simulink model "model_am_FOC"  (R2025a)
settings: Solver=ode3  StartTime=0.0  StopTime=2  FixedStep=0.0002  RelTol=1e-5  EnableMultiTasking=on
values from neighbouring files (symbols this model uses):
  I = 2.47    [parametres_AM.m]
  i2mN = i2mN2    [parametres_AM.m]
  J = 0.00096 * 5    (= 0.0048)    [parametres_AM.m]
  KI = R1 / (2 * sig * T1 * Kt)    (= 16.5280607989)    [parametres_AM.m]
  KrI = T2 / (2 * 2 * sig * T1)    (= 7.91437626335)    [parametres_AM.m]
  Krw = (J * (1 + sig2)) / (6 * sig * T1 * p^2 * Lh * i2mN)    [parametres_AM.m]
  Kt = 40    [parametres_AM.m]
  L1 = Lh + L1sig    (= 0.579)    [parametres_AM.m]
  L2 = L1    (= 0.579)    [parametres_AM.m]
  Lh = 0.56    [parametres_AM.m]
  M = 3.7    [parametres_AM.m]
  p = 2    [parametres_AM.m]
  R1 = 7.03    [parametres_AM.m]
  R2 = 3.44    [parametres_AM.m]
  sig = 1 - (Lh^2 / (L1 * L2))    (= 0.0645535599763)    [parametres_AM.m]
  T1 = L1 / R1    (= 0.0823613086771)    [parametres_AM.m]
  T2 = L2 / R2    (= 0.168313953488)    [parametres_AM.m]
  TiI = TrI / KrI    (= 0.0212668627176)    [parametres_AM.m]
  Tiw = Trw / Krw    [parametres_AM.m]
  Ulim = 380    [parametres_AM.m]
undefined symbols (not defined in the file or in its folder): sigbuilder_block
settings Model: Creator=Kajo  LastModifiedBy=emaka
settings SolverCC: AlgebraicLoopSolver=TrustRegion
settings DataIOCC: LimitDataPoints=on  SaveFormat=Array  SignalLoggingSaveFormat=ModelDataLogs  ReturnWorkspaceOutputs=off
settings OptimizationCC: ExpressionDepthLimit=2147483647.0  LifeSpan=inf
settings DebuggingCC: UnderspecifiedInitializationDetection=Classic  MergeDetectMultiDrivingBlocksExec=none  SolverPrmCheckMsg=warning  FcnCallInpInsideContextMsg=warning  UnconnectedInputMsg=warning  UnconnectedOutputMsg=warning  UnconnectedLineMsg=warning  StateNameClashWarn=warning  SFUnexpectedBacktrackingDiag=warning  SFNoUnconditionalDefaultTransitionDiag=warning  SFExecutionAtInitializationDiag=none  ArithmeticOperatorsInVariantConditions=warning
settings HardwareCC: ProdBitPerPointer=32.0  ProdBitPerSizeT=32.0  ProdBitPerPtrDiffT=32.0  ProdLargestAtomicFloat=None  ProdIntDivRoundTo=Undefined  ProdEndianess=Unspecified  ProdWordSize=32.0  ProdHWDeviceType=32-bit Generic
settings ModelReferenceCC: EnableRefExpFcnMdlSchedulingChecks=on  PropagateSignalLabelsOutOfModel=off
settings SFSimCC: SimUseLocalCustomCode=off  CustomCodeUndefinedFunction=UseInterfaceOnly
settings RTWCC: RTWUseLocalCustomCode=off  GPUComputeCapability=3.5
settings CodeAppCC: StateflowObjectComments=on
settings GRTTargetCC: TargetLangStandard=C89/C90 (ANSI)  CombineOutputUpdateFcns=off  GRTInterface=on
settings ConfigComp: CovMetricSettings=dw  CovSaveCumulativeToWorkspaceVar=on  CovSaveSingleToWorkspaceVar=on  CovExternalEMLEnable=off  CovSFcnEnable=off

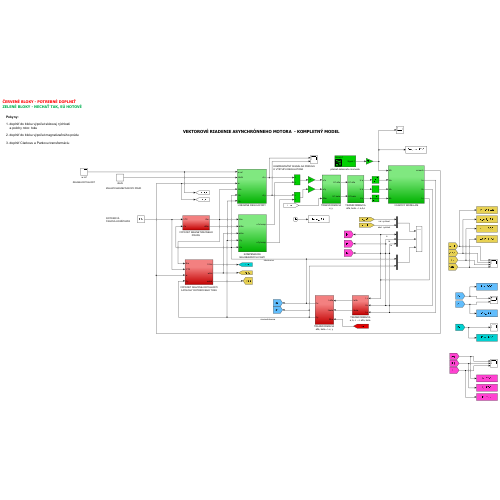
[thumbnail: Simulink's stored preview of the top-level diagram]
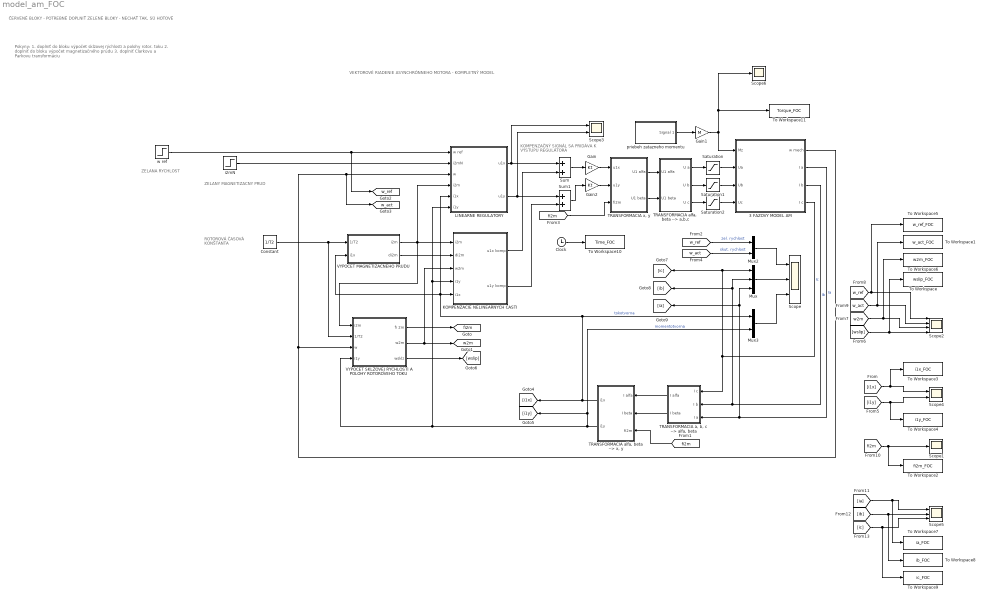
== system model_am_FOC ==
  note: Pokyny:
      |
      | 1. doplniť do bloku výpočet sklzovej rýchlosti
      | a polohy rotor. toku
      |
      | 2. doplniť do bloku výpočet magnetizačného prúdu
      |
      | 3. doplniť Clarkovu a Parkovu transformáciu
  note: ZELANA RYCHLOST
  note: KOMPENZAČNÝ SIGNÁL SA PRIDÁVA
      | K VÝSTUPU REGULÁTORA
  note: ROTOROVÁ
      | ČASOVÁ KONŠTANTA
  note: ČERVENÉ BLOKY - POTREBNÉ DOPLNIŤ
      | ZELENÉ BLOKY - NECHAŤ TAK, SÚ HOTOVÉ
  note: VEKTOROVÉ RIADENIE ASYNCHRÓNNEHO MOTORA - KOMPLETNÝ MODEL
  note: ZELANY MAGNETIZACNY PRUD
  3 FAZOVY MODEL AM : Subsystem
  Clock : Clock
  Constant : Constant  Value=1/T2
  Gain : Gain  Gain=Kt
  Gain1 : Gain  Gain=M
  Gain2 : Gain  Gain=Kt
  KOMPENZACIE NELINEARNYCH CASTI : Subsystem
  LINEARNE REGULATORY : Subsystem
  Mux : Mux  Inputs=3
  Mux2 : Mux  Inputs=2
  Mux3 : Mux  Inputs=2
  Saturation : Saturate  UpperLimit=Ulim  LowerLimit=-Ulim
  Saturation1 : Saturate  UpperLimit=Ulim  LowerLimit=-Ulim
  Saturation2 : Saturate  UpperLimit=Ulim  LowerLimit=-Ulim
  Scope : Scope  NumInputPorts=3
      settings: ActiveDisplayYMinimum=-13.916341130679911  ActiveDisplayYMaximum=125.24707017611922
  Scope1 : Scope
      settings: ActiveDisplayYMinimum=-1  ActiveDisplayYMaximum=1
  Scope2 : Scope  NumInputPorts=4
      settings: ActiveDisplayYMinimum=-1  ActiveDisplayYMaximum=1  DataLoggingVariableName=ScopeData3
  Scope3 : Scope  NumInputPorts=2
      settings: ActiveDisplayYMinimum=-0.016508812303007426  ActiveDisplayYMaximum=0.14857931072706687  DataLoggingVariableName=ScopeData4
  Scope4 : Scope  NumInputPorts=2
      settings: ActiveDisplayYMinimum=-1  ActiveDisplayYMaximum=1  DataLoggingVariableName=ScopeData5
  Scope5 : Scope  NumInputPorts=3
      settings: ActiveDisplayYMinimum=-1  ActiveDisplayYMaximum=1  DataLoggingVariableName=ScopeData6
  Scope6 : Scope
      settings: ActiveDisplayYMinimum=-1  ActiveDisplayYMaximum=1  DataLoggingVariableName=ScopeData7
  Sum : Sum
  Sum1 : Sum
  "TRANSFORMACIA a, b, c  --> alfa, beta " : Subsystem
  "TRANSFORMACIA alfa, beta --> a,b,c" : Subsystem
  "TRANSFORMACIA alfa, beta --> x, y" : Subsystem
  "TRANSFORMACIA x, y " : Subsystem
  To Workspace : ToWorkspace  VariableName=wslip_FOC  SampleTime=-1
  To Workspace1 : ToWorkspace  VariableName=w_act_FOC  SampleTime=-1
  To Workspace10 : ToWorkspace  VariableName=Time_FOC  SampleTime=-1
  To Workspace11 : ToWorkspace  VariableName=Torque_FOC  SampleTime=-1
  To Workspace2 : ToWorkspace  VariableName=fi2m_FOC  SampleTime=-1
  To Workspace3 : ToWorkspace  VariableName=i1x_FOC  SampleTime=-1
  To Workspace4 : ToWorkspace  VariableName=i1y_FOC  SampleTime=-1
  To Workspace5 : ToWorkspace  VariableName=w_ref_FOC  SampleTime=-1
  To Workspace6 : ToWorkspace  VariableName=w2m_FOC  SampleTime=-1
  To Workspace7 : ToWorkspace  VariableName=ia_FOC  SampleTime=-1
  To Workspace8 : ToWorkspace  VariableName=ib_FOC  SampleTime=-1
  To Workspace9 : ToWorkspace  VariableName=ic_FOC  SampleTime=-1
  VYPOCET MAGNETIZACNEHO PRUDU : Subsystem
  VYPOCET SKLZOVEJ RYCHLOSTI A POLOHY ROTOROVEHO TOKU : Subsystem
  i2mN : Step  Time=0  After=i2mN  SampleTime=0
  priebeh zatazneho momentu : Subsystem  Tag=STV Subsys  LoadFcn=sigbuilder_block('load');  StartFcn=sigbuilder_block('start');  StopFcn=sigbuilder_block('stop');  ClipboardFcn=sigbuilder_block('clipboard');  mask(Sigbuilder block){tuvar=[0:10]}
      mask help: Simulink:masks:SigbuilderBlock_MD
      mask init:
      | if ~strcmp(get_param(bdroot(gcbh),'SimulationStatus'),'stopped') tuvar = sigbuilder_block('maskInit'); end
      settings: CopyFcn=sigbuilder_block('copy');  DeleteFcn=sigbuilder_block('delete');  ModelCloseFcn=sigbuilder_block('modelClose');  PreSaveFcn=sigbuilder_block('preSave');  PauseFcn=sigbuilder_block('pause');  ContinueFcn=sigbuilder_block('continue');  NameChangeFcn=sigbuilder_block('namechange');  OpenFcn=sigbuilder_block('open',[436.5 297.75 1045.5 630 ]);  CloseFcn=sigbuilder_block('close');
      mask Display: plot(0, 0, 100, 100,[2, 2, 32, 32, 2], [68, 8, 8, 68, 68],[32, 2], [38, 38], [32, 19, 2],[53, 60, 44], [32, 17, 17, 2],[16, 16, 31, 31]);txt = getActiveGroup(gcbh);text(2, 100, txt,'verticalAlignment', 'top');
  w ref : Step  Time=0.4  After=70  SampleTime=0
  tag scope: fi2m=global, w2m=global, w_act=global, w_ref=global
  wires:
  priebeh zatazneho momentu/1(Signal 1) -> Gain1/1
  Gain1/1 -> 3 FAZOVY MODEL AM/1(Mz), Scope6/1, To Workspace11/1
  LINEARNE REGULATORY/1(u1x) -> Sum/1, Scope3/1
  LINEARNE REGULATORY/2(u1y) -> Scope3/2, Sum1/1
  KOMPENZACIE NELINEARNYCH CASTI/1(u1x komp) -> Sum/2
  KOMPENZACIE NELINEARNYCH CASTI/2(u1y komp) -> Sum1/2
  "TRANSFORMACIA a, b, c  --> alfa, beta "/1(I alfa) -> "TRANSFORMACIA alfa, beta --> x, y"/1(I alfa)
  "TRANSFORMACIA a, b, c  --> alfa, beta "/2(I beta) -> "TRANSFORMACIA alfa, beta --> x, y"/2(I beta)
  3 FAZOVY MODEL AM/1(w mech) -> [w_act], LINEARNE REGULATORY/3(w), VYPOCET SKLZOVEJ RYCHLOSTI A POLOHY ROTOROVEHO TOKU/3(w)
  i2mN/1 -> LINEARNE REGULATORY/2(i2mN)
  3 FAZOVY MODEL AM/4(I c) -> Mux/1, [ic], "TRANSFORMACIA a, b, c  --> alfa, beta "/1(I c)  "Ic"
  3 FAZOVY MODEL AM/3(I b) -> Mux/2, [ib], "TRANSFORMACIA a, b, c  --> alfa, beta "/2(I b)  "Ib"
  3 FAZOVY MODEL AM/2(I a) -> [ia], Mux/3, "TRANSFORMACIA a, b, c  --> alfa, beta "/3(I a)  "Ia"
  Constant/1 -> VYPOCET SKLZOVEJ RYCHLOSTI A POLOHY ROTOROVEHO TOKU/2(1/T2), VYPOCET MAGNETIZACNEHO PRUDU/1(1/T2)
  VYPOCET MAGNETIZACNEHO PRUDU/1(i2m) -> LINEARNE REGULATORY/4(i2m), VYPOCET SKLZOVEJ RYCHLOSTI A POLOHY ROTOROVEHO TOKU/1(i2m), KOMPENZACIE NELINEARNYCH CASTI/1(i2m)
  VYPOCET MAGNETIZACNEHO PRUDU/2(di2m) -> KOMPENZACIE NELINEARNYCH CASTI/2(di2m)
  Gain/1 -> "TRANSFORMACIA x, y "/1(u1x)
  Gain2/1 -> "TRANSFORMACIA x, y "/2(u1y)
  "TRANSFORMACIA x, y "/1(U1 alfa) -> "TRANSFORMACIA alfa, beta --> a,b,c"/1(U1 alfa)
  "TRANSFORMACIA x, y "/2(U1 beta) -> "TRANSFORMACIA alfa, beta --> a,b,c"/2(U1 beta)
  "TRANSFORMACIA alfa, beta --> a,b,c"/1(U a) -> Saturation/1
  "TRANSFORMACIA alfa, beta --> a,b,c"/2(U b) -> Saturation1/1
  "TRANSFORMACIA alfa, beta --> a,b,c"/3(U c) -> Saturation2/1
  Saturation/1 -> 3 FAZOVY MODEL AM/2(Ua)
  Saturation1/1 -> 3 FAZOVY MODEL AM/3(Ub)
  Saturation2/1 -> 3 FAZOVY MODEL AM/4(Uc)
  Sum/1 -> Gain/1
  Sum1/1 -> Gain2/1
  "TRANSFORMACIA alfa, beta --> x, y"/2(i1y) -> [i1y], Mux3/2, KOMPENZACIE NELINEARNYCH CASTI/4(i1y), LINEARNE REGULATORY/6(i1y), VYPOCET SKLZOVEJ RYCHLOSTI A POLOHY ROTOROVEHO TOKU/4(i1y)  "momentotvorna"
  VYPOCET SKLZOVEJ RYCHLOSTI A POLOHY ROTOROVEHO TOKU/2(w2m) -> KOMPENZACIE NELINEARNYCH CASTI/3(w2m), [w2m]
  "TRANSFORMACIA alfa, beta --> x, y"/1(i1x) -> [i1x], LINEARNE REGULATORY/5(i1x), VYPOCET MAGNETIZACNEHO PRUDU/2(i1x), KOMPENZACIE NELINEARNYCH CASTI/5(i1x), Mux3/1  "tokotvorna"
  w ref/1 -> LINEARNE REGULATORY/1(w ref), [w_ref]
  VYPOCET SKLZOVEJ RYCHLOSTI A POLOHY ROTOROVEHO TOKU/1(fi 2m) -> [fi2m]
  [fi2m] -> "TRANSFORMACIA alfa, beta --> x, y"/3(fi2m)
  [fi2m] -> "TRANSFORMACIA x, y "/3("fi2m ")
  Mux2/1 -> Scope/1
  [w_ref] -> Mux2/1  "zel. rychlost"
  [w_act] -> Mux2/2  "skut. rychlost"
  Mux3/1 -> Scope/3
  Mux/1 -> Scope/2
  [i1x] -> To Workspace3/1, Scope4/1
  [i1y] -> To Workspace4/1, Scope4/2
  VYPOCET SKLZOVEJ RYCHLOSTI A POLOHY ROTOROVEHO TOKU/3(wsklz) -> [wslip]
  [wslip] -> To Workspace/1, Scope2/4
  [w2m] -> To Workspace6/1, Scope2/3
  [w_ref] -> To Workspace5/1, Scope2/1
  [w_act] -> To Workspace1/1, Scope2/2
  [fi2m] -> To Workspace2/1, Scope1/1
  [ia] -> To Workspace7/1, Scope5/1
  [ib] -> To Workspace8/1, Scope5/2
  [ic] -> To Workspace9/1, Scope5/3
  Clock/1 -> To Workspace10/1

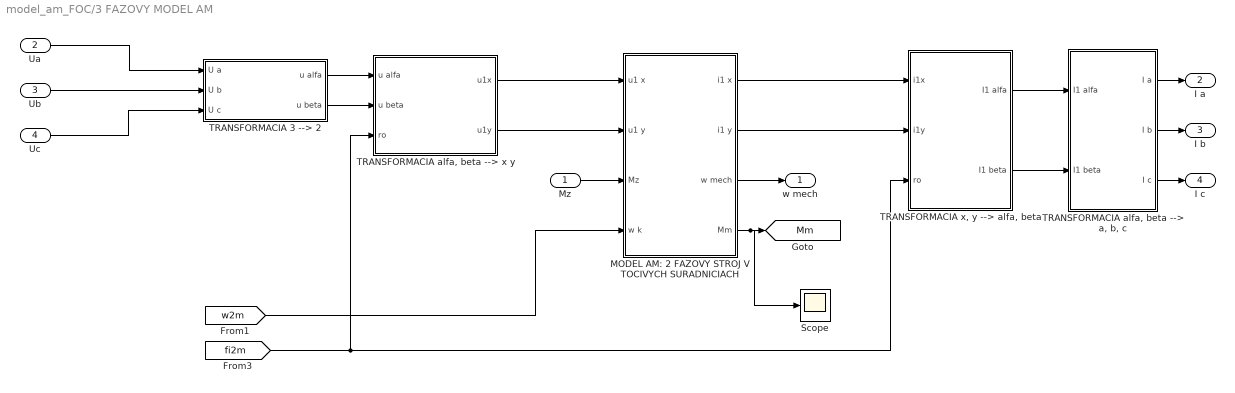
== system model_am_FOC/3 FAZOVY MODEL AM ==
  Mz : Inport
  Ua : Inport  Port=2
  Ub : Inport  Port=3
  Uc : Inport  Port=4
  MODEL AM: 2 FAZOVY STROJ V TOCIVYCH SURADNICIACH : Subsystem
  Scope : Scope
      settings: ActiveDisplayYMinimum=-2.9719517266428888  ActiveDisplayYMaximum=3.6440018137289671  DataLoggingVariableName=ScopeData2
  "TRANSFORMACIA alfa, beta --> x y" : Subsystem
  TRANSFORMACIA 3 --> 2 : Subsystem
  "TRANSFORMACIA alfa, beta --> a, b, c" : Subsystem
  "TRANSFORMACIA x, y --> alfa, beta" : Subsystem
  w mech : Outport  VectorParamsAs1DForOutWhenUnconnected=off
  I a : Outport  Port=2  VectorParamsAs1DForOutWhenUnconnected=off
  I b : Outport  Port=3  VectorParamsAs1DForOutWhenUnconnected=off
  I c : Outport  Port=4  VectorParamsAs1DForOutWhenUnconnected=off
  tag scope: Mm=global
  wires:
  TRANSFORMACIA 3 --> 2/1(u alfa) -> "TRANSFORMACIA alfa, beta --> x y"/1(u alfa)
  TRANSFORMACIA 3 --> 2/2(u beta) -> "TRANSFORMACIA alfa, beta --> x y"/2(u beta)
  "TRANSFORMACIA alfa, beta --> x y"/1(u1x) -> MODEL AM: 2 FAZOVY STROJ V TOCIVYCH SURADNICIACH/1(u1 x)
  "TRANSFORMACIA alfa, beta --> x y"/2(u1y) -> MODEL AM: 2 FAZOVY STROJ V TOCIVYCH SURADNICIACH/2(u1 y)
  "TRANSFORMACIA x, y --> alfa, beta"/1(I1 alfa) -> "TRANSFORMACIA alfa, beta --> a, b, c"/1(I1 alfa)
  "TRANSFORMACIA x, y --> alfa, beta"/2(I1 beta) -> "TRANSFORMACIA alfa, beta --> a, b, c"/2(I1 beta)
  "TRANSFORMACIA alfa, beta --> a, b, c"/1(I a) -> I a/1
  "TRANSFORMACIA alfa, beta --> a, b, c"/2(I b) -> I b/1
  "TRANSFORMACIA alfa, beta --> a, b, c"/3(I c) -> I c/1
  Ua/1 -> TRANSFORMACIA 3 --> 2/1(U a)
  Ub/1 -> TRANSFORMACIA 3 --> 2/2(U b)
  Uc/1 -> TRANSFORMACIA 3 --> 2/3(U c)
  Mz/1 -> MODEL AM: 2 FAZOVY STROJ V TOCIVYCH SURADNICIACH/3(Mz)
  MODEL AM: 2 FAZOVY STROJ V TOCIVYCH SURADNICIACH/1(i1 x) -> "TRANSFORMACIA x, y --> alfa, beta"/1(i1x)
  MODEL AM: 2 FAZOVY STROJ V TOCIVYCH SURADNICIACH/2(i1 y) -> "TRANSFORMACIA x, y --> alfa, beta"/2(i1y)
  MODEL AM: 2 FAZOVY STROJ V TOCIVYCH SURADNICIACH/3(w mech) -> w mech/1
  [fi2m] -> "TRANSFORMACIA x, y --> alfa, beta"/3("ro "), "TRANSFORMACIA alfa, beta --> x y"/3(ro)
  [w2m] -> MODEL AM: 2 FAZOVY STROJ V TOCIVYCH SURADNICIACH/4(w k)
  MODEL AM: 2 FAZOVY STROJ V TOCIVYCH SURADNICIACH/4(Mm) -> Scope/1, [Mm]

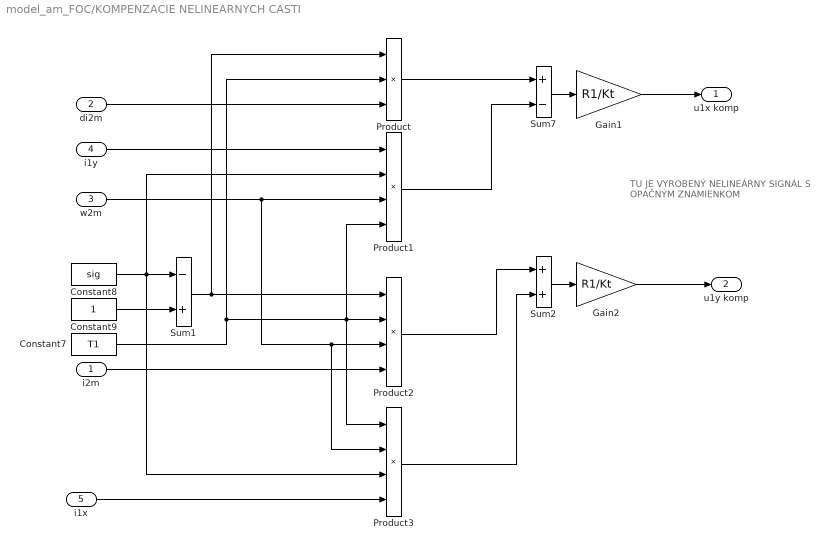
== system model_am_FOC/KOMPENZACIE NELINEARNYCH CASTI ==
  note: TU JE VYROBENÝ NELINEÁRNY SIGNÁL
      | S OPAČNÝM ZNAMIENKOM
  i2m : Inport
  di2m : Inport  Port=2
  w2m : Inport  Port=3
  i1y : Inport  Port=4
  i1x : Inport  Port=5
  Constant7 : Constant  Value=T1
  Constant8 : Constant  Value=sig
  Constant9 : Constant
  Gain1 : Gain  Gain=R1/Kt
  Gain2 : Gain  Gain=R1/Kt
  Product : Product  Inputs=3  RndMeth=Zero
  Product1 : Product  Inputs=4  RndMeth=Zero
  Product2 : Product  Inputs=4  RndMeth=Zero
  Product3 : Product  Inputs=4  RndMeth=Zero
  Sum1 : Sum  Inputs=-+
  Sum2 : Sum
  Sum7 : Sum  Inputs=+-
  u1x komp : Outport  VectorParamsAs1DForOutWhenUnconnected=off
  u1y komp : Outport  Port=2  VectorParamsAs1DForOutWhenUnconnected=off
  wires:
  Sum7/1 -> Gain1/1
  Sum2/1 -> Gain2/1
  Product/1 -> Sum7/1
  Product1/1 -> Sum7/2
  Product2/1 -> Sum2/1
  Product3/1 -> Sum2/2
  Constant9/1 -> Sum1/2
  Sum1/1 -> Product/1, Product2/1
  Constant7/1 -> Product/2, Product2/2, Product1/4, Product3/1
  di2m/1 -> Product/3
  i2m/1 -> Product2/4
  w2m/1 -> Product1/3, Product2/3, Product3/2
  i1y/1 -> Product1/1
  i1x/1 -> Product3/4
  Constant8/1 -> Sum1/1, Product1/2, Product3/3
  Gain1/1 -> u1x komp/1
  Gain2/1 -> u1y komp/1

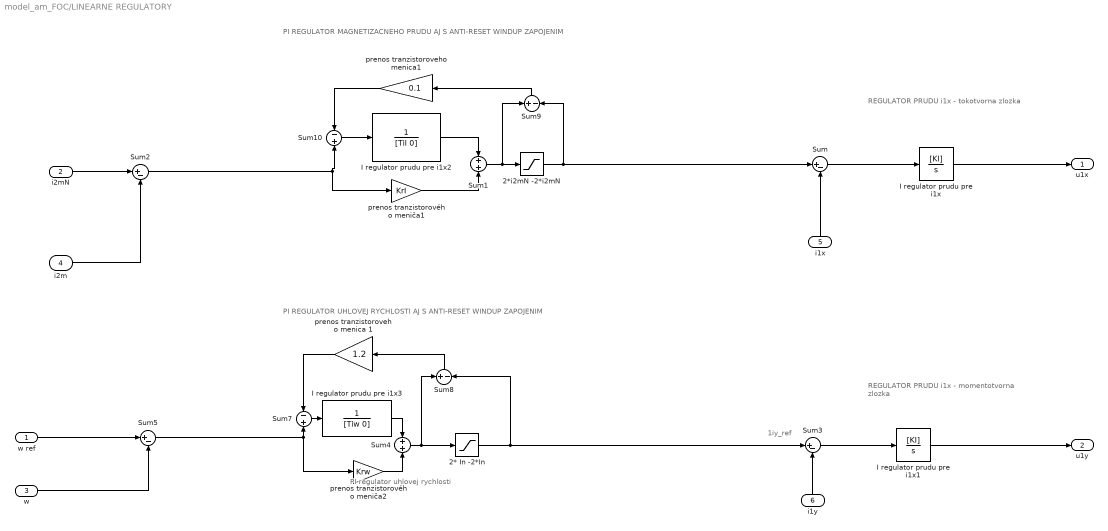
== system model_am_FOC/LINEARNE REGULATORY ==
  note: REGULATOR PRUDU
      | i1x - tokotvorna zlozka
  note: PI REGULATOR MAGNETIZACNEHO PRUDU
      | AJ S ANTI-RESET WINDUP ZAPOJENIM
  note: 1iy_ref
  note: PI regulator
      | uhlovej rychlosti
  note: PI REGULATOR UHLOVEJ RYCHLOSTI
      | AJ S ANTI-RESET WINDUP ZAPOJENIM
  note: REGULATOR PRUDU
      | i1x - momentotvorna zlozka
  w ref : Inport
  i2mN : Inport  Port=2
  w : Inport  Port=3
  i2m : Inport  Port=4
  i1x : Inport  Port=5
  i1y : Inport  Port=6
  2* In -2*In : Saturate  UpperLimit=I*1.5  LowerLimit=-I*1.5
  2*i2mN -2*i2mN : Saturate  UpperLimit=1.5*i2mN  LowerLimit=-1.5*i2mN
  I regulator prudu pre i1x : TransferFcn  Numerator=[KI]  Denominator=[1 0]
  I regulator prudu pre i1x1 : TransferFcn  Numerator=[KI]  Denominator=[1 0]
  I regulator prudu pre i1x2 : TransferFcn  Denominator=[TiI 0]
  I regulator prudu pre i1x3 : TransferFcn  Denominator=[Tiw 0]
  Sum{,2..3,5} (4 alike) : Sum  Inputs=|+-
  Sum1 : Sum
  Sum10 : Sum  Inputs=-+
  Sum4 : Sum
  Sum7 : Sum  Inputs=-+
  Sum8 : Sum  Inputs=+-
  Sum9 : Sum  Inputs=+-
  prenos tranzistoroveho menica 1 : Gain  Gain=1.2
  prenos tranzistoroveho menica1 : Gain  Gain=0.1
  prenos tranzistorového meniča1 : Gain  Gain=KrI
  prenos tranzistorového meniča2 : Gain  Gain=Krw
  u1x : Outport  VectorParamsAs1DForOutWhenUnconnected=off
  u1y : Outport  Port=2  VectorParamsAs1DForOutWhenUnconnected=off
  wires:
  w ref/1 -> Sum5/1
  i1x/1 -> Sum/2
  i1y/1 -> Sum3/2
  w/1 -> Sum5/2
  i2mN/1 -> Sum2/1
  i2m/1 -> Sum2/2
  2* In -2*In/1 -> Sum8/2, Sum3/1
  I regulator prudu pre i1x/1 -> u1x/1
  I regulator prudu pre i1x1/1 -> u1y/1
  Sum/1 -> I regulator prudu pre i1x/1
  Sum3/1 -> I regulator prudu pre i1x1/1
  Sum1/1 -> 2*i2mN -2*i2mN/1, Sum9/1
  Sum9/1 -> prenos tranzistoroveho menica1/1
  Sum2/1 -> prenos tranzistorového meniča1/1, Sum10/2
  prenos tranzistorového meniča1/1 -> Sum1/2
  I regulator prudu pre i1x2/1 -> Sum1/1
  prenos tranzistoroveho menica1/1 -> Sum10/1
  Sum10/1 -> I regulator prudu pre i1x2/1
  2*i2mN -2*i2mN/1 -> Sum/1, Sum9/2
  Sum5/1 -> prenos tranzistorového meniča2/1, Sum7/2
  Sum7/1 -> I regulator prudu pre i1x3/1
  prenos tranzistorového meniča2/1 -> Sum4/2
  I regulator prudu pre i1x3/1 -> Sum4/1
  Sum8/1 -> prenos tranzistoroveho menica 1/1
  Sum4/1 -> 2* In -2*In/1, Sum8/1
  prenos tranzistoroveho menica 1/1 -> Sum7/1

== system model_am_FOC/TRANSFORMACIA a, b, c  --> alfa, beta  ==
  I c : Inport
  I b : Inport  Port=2
  I a : Inport  Port=3
  Gain : Gain  Gain=1/sqrt(3)
  Sum : Sum  Inputs=|+-
  I alfa : Outport  VectorParamsAs1DForOutWhenUnconnected=off
  I beta : Outport  Port=2  VectorParamsAs1DForOutWhenUnconnected=off
  wires:
  I b/1 -> Sum/1
  I c/1 -> Sum/2
  Sum/1 -> Gain/1
  Gain/1 -> I beta/1
  I a/1 -> I alfa/1

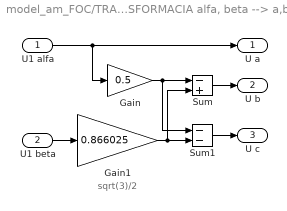
== system model_am_FOC/TRANSFORMACIA alfa, beta --> a,b,c ==
  note: sqrt(3)/2
  U1 alfa : Inport
  U1 beta : Inport  Port=2
  Gain : Gain  Gain=0.5
  Gain1 : Gain  Gain=0.866025
  Sum : Sum  Inputs=-+
  Sum1 : Sum  Inputs=--
  U a : Outport  VectorParamsAs1DForOutWhenUnconnected=off
  U b : Outport  Port=2  VectorParamsAs1DForOutWhenUnconnected=off
  U c : Outport  Port=3  VectorParamsAs1DForOutWhenUnconnected=off
  wires:
  Sum1/1 -> U c/1
  Gain1/1 -> Sum1/2, Sum/2
  U1 beta/1 -> Gain1/1
  Sum/1 -> U b/1
  Gain/1 -> Sum1/1, Sum/1
  U1 alfa/1 -> U a/1, Gain/1

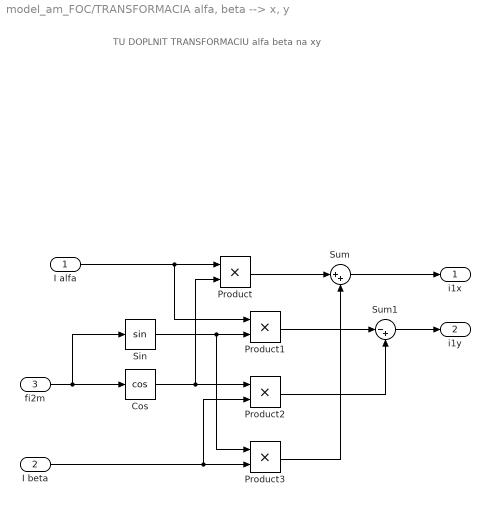
== system model_am_FOC/TRANSFORMACIA alfa, beta --> x, y ==
  note: TU DOPLNIT TRANSFORMACIU
      | alfa beta na xy
  I alfa : Inport
  I beta : Inport  Port=2
  fi2m : Inport  Port=3
  Cos : Trigonometry  Operator=cos
  Product{,1..3} (4 alike) : Product
  Sin : Trigonometry
  Sum : Sum  Inputs=|++
  Sum1 : Sum  Inputs=|-+
  i1x : Outport  VectorParamsAs1DForOutWhenUnconnected=off
  i1y : Outport  Port=2  VectorParamsAs1DForOutWhenUnconnected=off
  wires:
  I alfa/1 -> Product1/1, Product/1
  Product/1 -> Sum/1
  fi2m/1 -> Sin/1, Cos/1
  Sin/1 -> Product3/1, Product1/2
  Cos/1 -> Product2/1, Product/2
  I beta/1 -> Product3/2, Product2/2
  Product3/1 -> Sum/2
  Product1/1 -> Sum1/1
  Sum/1 -> i1x/1
  Sum1/1 -> i1y/1
  Product2/1 -> Sum1/2

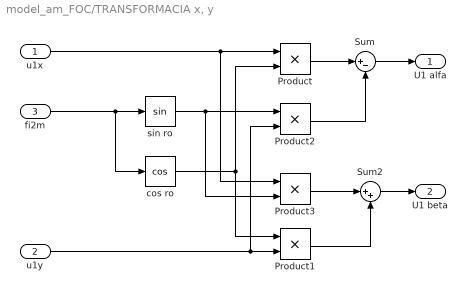
== system model_am_FOC/TRANSFORMACIA x, y  ==
  u1x : Inport
  u1y : Inport  Port=2
  "fi2m " : Inport  Port=3
  Product{,1..3} (4 alike) : Product  RndMeth=Zero
  Sum : Sum  Inputs=|+-
  Sum2 : Sum  Inputs=|++
  cos ro : Trigonometry  Operator=cos
  sin ro : Trigonometry
  U1 alfa : Outport  VectorParamsAs1DForOutWhenUnconnected=off
  U1 beta : Outport  Port=2  VectorParamsAs1DForOutWhenUnconnected=off
  wires:
  Product1/1 -> Sum2/2
  Product3/1 -> Sum2/1
  Product2/1 -> Sum/2
  Product/1 -> Sum/1
  u1y/1 -> Product2/2, Product1/2
  sin ro/1 -> Product3/2, Product2/1
  cos ro/1 -> Product1/1, Product/2
  u1x/1 -> Product/1, Product3/1
  Sum2/1 -> U1 beta/1
  Sum/1 -> U1 alfa/1
  "fi2m "/1 -> cos ro/1, sin ro/1

== system model_am_FOC/VYPOCET MAGNETIZACNEHO PRUDU ==
  note: TU DOPLNIT VYPOCET
      | MAGNETIZACNEHO PRUDU
  1/T2 : Inport
  i1x : Inport  Port=2
  Integrator : Integrator
  Product : Product
  Sum : Sum  Inputs=|+-
  i2m : Outport  VectorParamsAs1DForOutWhenUnconnected=off
  di2m : Outport  Port=2  VectorParamsAs1DForOutWhenUnconnected=off
  wires:
  i1x/1 -> Sum/1
  1/T2/1 -> Product/2
  Product/1 -> di2m/1, Integrator/1
  Sum/1 -> Product/1
  Integrator/1 -> i2m/1, Sum/2

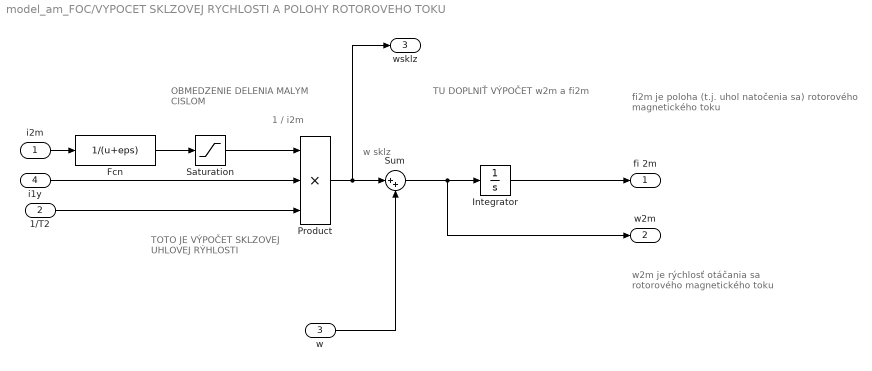
== system model_am_FOC/VYPOCET SKLZOVEJ RYCHLOSTI A POLOHY ROTOROVEHO TOKU ==
  note: TOTO JE VÝPOČET
      | SKLZOVEJ UHLOVEJ RÝHLOSTI
  note: TU DOPLNIŤ
      | VÝPOČET w2m a fi2m
  note: 1 / i2m
  note: w sklz
  note: OBMEDZENIE
      | DELENIA
      | MALYM CISLOM
  note: w2m je rýchlosť
      | otáčania sa rotorového
      | magnetického toku
  note: fi2m je poloha (t.j. uhol natočenia sa) rotorového
      | magnetického toku
  i2m : Inport
  1/T2 : Inport  Port=2
  w : Inport  Port=3
  i1y : Inport  Port=4
  Fcn : Fcn  Expr=1/(u+eps)
  Integrator : Integrator
  Product : Product  Inputs=3  RndMeth=Zero
  Saturation : Saturate  UpperLimit=300  LowerLimit=-300
  Sum : Sum  Inputs=|++
  fi 2m : Outport  VectorParamsAs1DForOutWhenUnconnected=off
  w2m : Outport  Port=2  VectorParamsAs1DForOutWhenUnconnected=off
  wsklz : Outport  Port=3
  wires:
  1/T2/1 -> Product/3
  i2m/1 -> Fcn/1
  Fcn/1 -> Saturation/1
  Product/1 -> wsklz/1, Sum/1
  w/1 -> Sum/2
  Saturation/1 -> Product/1
  i1y/1 -> Product/2
  Sum/1 -> w2m/1, Integrator/1
  Integrator/1 -> fi 2m/1

== system model_am_FOC/priebeh zatazneho momentu ==
  Demux : Demux  Tag=STV Demux  Outputs=1
      settings: DisplayOption=none
  FromWs : FromWorkspace  Tag=STV FromWs  VariableName=tuvar
      SigBuilderData=|
      | common.afterFinalStr = 'Extrapolate'
      | common.sampleTime = 0
      | dataSet.timeRange = [0 5]
      | dataSet.name = 'Group 1'
      | sbobj.Groups.Name = 'Group 1'
      | sbobj.Groups.Signals.Name = 'Signal 1'
      | sbobj.Groups.Signals.XData = [0 1.2 1.2 5]
      | sbobj.Groups.Signals.YData = [0 0 0.5 0.5]
      | sbobj.Groups.TimeRange = [0 5]
  Signal 1 : Outport  Tag=STV Outport  VectorParamsAs1DForOutWhenUnconnected=off
  wires:
  Demux/1 -> Signal 1/1
  FromWs/1 -> Demux/1

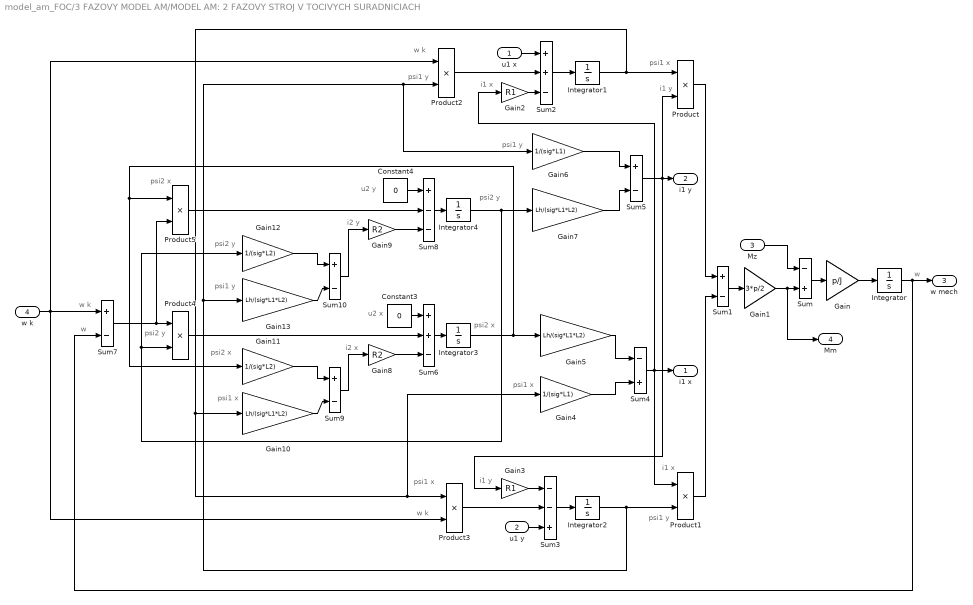
== system model_am_FOC/3 FAZOVY MODEL AM/MODEL AM: 2 FAZOVY STROJ V TOCIVYCH SURADNICIACH ==
  note: w
  note: psi1 x
  note: i1 y
  note: psi1 y
  note: i1 x
  note: i1 x
  note: w k
  note: psi1 y
  note: i1 y
  note: w k
  note: psi1 x
  note: psi1 x
  note: psi2 x
  note: psi1 y
  note: psi2 y
  note: u2 x
  note: i2 x
  note: psi2 y
  note: w
  note: i2 y
  note: u2 y
  note: psi2 x
  note: psi1 x
  note: psi2 x
  note: psi2 y
  note: psi1 y
  note: w k
  u1 x : Inport
  u1 y : Inport  Port=2
  Mz : Inport  Port=3
  w k : Inport  Port=4
  Constant3 : Constant  Value=0
  Constant4 : Constant  Value=0
  Gain : Gain  Gain=p/J
  Gain1 : Gain  Gain=3*p/2
  Gain{5,7,10,13} (4 alike) : Gain  Gain=Lh/(sig*L1*L2)
  Gain11 : Gain  Gain=1/(sig*L2)
  Gain12 : Gain  Gain=1/(sig*L2)
  Gain2 : Gain  Gain=R1
  Gain3 : Gain  Gain=R1
  Gain4 : Gain  Gain=1/(sig*L1)
  Gain6 : Gain  Gain=1/(sig*L1)
  Gain8 : Gain  Gain=R2
  Gain9 : Gain  Gain=R2
  Integrator{,1..4} (5 alike) : Integrator
  Product{,1..5} (6 alike) : Product  RndMeth=Zero
  Sum : Sum  Inputs=-+
  Sum{1,5,7,9..10} (5 alike) : Sum  Inputs=+-
  Sum2 : Sum  Inputs=++-
  Sum3 : Sum  Inputs=--+
  Sum4 : Sum  Inputs=-+
  Sum6 : Sum  Inputs=++-
  Sum8 : Sum  Inputs=+--
  i1 x : Outport  VectorParamsAs1DForOutWhenUnconnected=off
  i1 y : Outport  Port=2  VectorParamsAs1DForOutWhenUnconnected=off
  w mech : Outport  Port=3  VectorParamsAs1DForOutWhenUnconnected=off
  Mm : Outport  Port=4  VectorParamsAs1DForOutWhenUnconnected=off
  wires:
  Gain/1 -> Integrator/1
  Sum/1 -> Gain/1
  Sum1/1 -> Gain1/1
  Gain1/1 -> Sum/2, Mm/1
  Integrator/1 -> Sum7/2, w mech/1
  Product/1 -> Sum1/1
  Product1/1 -> Sum1/2
  Integrator1/1 -> Product/1, Gain10/1, Product3/1, Gain4/1
  Integrator2/1 -> Product1/2, Gain13/1, Product2/2, Gain6/1
  Sum2/1 -> Integrator1/1
  Sum3/1 -> Integrator2/1
  Gain2/1 -> Sum2/3
  Product2/1 -> Sum2/2
  u1 x/1 -> Sum2/1
  Product3/1 -> Sum3/2
  Sum4/1 -> Gain2/1, i1 x/1, Product1/1
  Gain5/1 -> Sum4/1
  Gain6/1 -> Sum5/1
  Sum5/1 -> Product/2, Gain3/1, i1 y/1
  Gain7/1 -> Sum5/2
  Integrator3/1 -> Gain5/1, Product5/1, Gain11/1
  Integrator4/1 -> Gain7/1, Product4/2, Gain12/1
  Sum6/1 -> Integrator3/1
  Constant3/1 -> Sum6/1
  Gain8/1 -> Sum6/3
  Product4/1 -> Sum6/2
  Sum7/1 -> Product5/2, Product4/1
  Sum8/1 -> Integrator4/1
  Gain9/1 -> Sum8/3
  Constant4/1 -> Sum8/1
  Product5/1 -> Sum8/2
  Sum9/1 -> Gain8/1
  Gain10/1 -> Sum9/2
  Gain11/1 -> Sum9/1
  Sum10/1 -> Gain9/1
  Gain12/1 -> Sum10/1
  Gain13/1 -> Sum10/2
  w k/1 -> Product3/2, Product2/1, Sum7/1
  Gain4/1 -> Sum4/2
  u1 y/1 -> Sum3/3
  Gain3/1 -> Sum3/1
  Mz/1 -> Sum/1

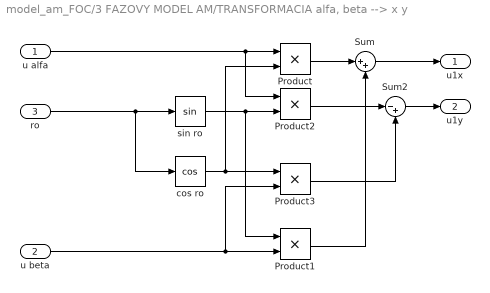
== system model_am_FOC/3 FAZOVY MODEL AM/TRANSFORMACIA alfa, beta --> x y ==
  u alfa : Inport
  u beta : Inport  Port=2
  ro : Inport  Port=3
  Product{,1..3} (4 alike) : Product  RndMeth=Zero
  Sum : Sum  Inputs=|++
  Sum2 : Sum  Inputs=|-+
  cos ro : Trigonometry  Operator=cos
  sin ro : Trigonometry
  u1x : Outport  VectorParamsAs1DForOutWhenUnconnected=off
  u1y : Outport  Port=2  VectorParamsAs1DForOutWhenUnconnected=off
  wires:
  Product3/1 -> Sum2/2
  Sum2/1 -> u1y/1
  Product2/1 -> Sum2/1
  Sum/1 -> u1x/1
  Product1/1 -> Sum/2
  Product/1 -> Sum/1
  u beta/1 -> Product1/2, Product3/2
  sin ro/1 -> Product2/2, Product1/1
  u alfa/1 -> Product/1, Product2/1
  cos ro/1 -> Product3/1, Product/2
  ro/1 -> sin ro/1, cos ro/1

== system model_am_FOC/3 FAZOVY MODEL AM/TRANSFORMACIA 3 --> 2 ==
  U a : Inport
  U b : Inport  Port=2
  U c : Inport  Port=3
  1/sqrt(3) : Gain  Gain=0.57735
  Sum : Sum  Inputs=|+-
  u alfa : Outport  VectorParamsAs1DForOutWhenUnconnected=off
  u beta : Outport  Port=2  VectorParamsAs1DForOutWhenUnconnected=off
  wires:
  U b/1 -> Sum/1
  U c/1 -> Sum/2
  1/sqrt(3)/1 -> u beta/1
  U a/1 -> u alfa/1
  Sum/1 -> 1/sqrt(3)/1

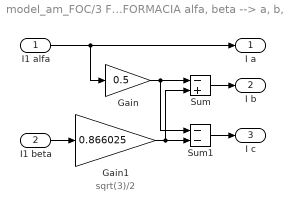
== system model_am_FOC/3 FAZOVY MODEL AM/TRANSFORMACIA alfa, beta --> a, b, c ==
  note: sqrt(3)/2
  I1 alfa : Inport
  I1 beta : Inport  Port=2
  Gain : Gain  Gain=0.5
  Gain1 : Gain  Gain=0.866025
  Sum : Sum  Inputs=-+
  Sum1 : Sum  Inputs=--
  I a : Outport  VectorParamsAs1DForOutWhenUnconnected=off
  I b : Outport  Port=2  VectorParamsAs1DForOutWhenUnconnected=off
  I c : Outport  Port=3  VectorParamsAs1DForOutWhenUnconnected=off
  wires:
  Sum1/1 -> I c/1
  Gain1/1 -> Sum1/2, Sum/2
  I1 beta/1 -> Gain1/1
  Sum/1 -> I b/1
  Gain/1 -> Sum1/1, Sum/1
  I1 alfa/1 -> I a/1, Gain/1

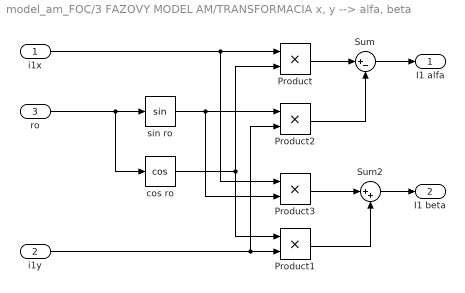
== system model_am_FOC/3 FAZOVY MODEL AM/TRANSFORMACIA x, y --> alfa, beta ==
  i1x : Inport
  i1y : Inport  Port=2
  "ro " : Inport  Port=3
  Product{,1..3} (4 alike) : Product  RndMeth=Zero
  Sum : Sum  Inputs=|+-
  Sum2 : Sum  Inputs=|++
  cos ro : Trigonometry  Operator=cos
  sin ro : Trigonometry
  I1 alfa : Outport  VectorParamsAs1DForOutWhenUnconnected=off
  I1 beta : Outport  Port=2  VectorParamsAs1DForOutWhenUnconnected=off
  wires:
  Product1/1 -> Sum2/2
  Product3/1 -> Sum2/1
  Product2/1 -> Sum/2
  Product/1 -> Sum/1
  i1y/1 -> Product2/2, Product1/2
  sin ro/1 -> Product3/2, Product2/1
  cos ro/1 -> Product1/1, Product/2
  i1x/1 -> Product/1, Product3/1
  Sum2/1 -> I1 beta/1
  Sum/1 -> I1 alfa/1
  "ro "/1 -> cos ro/1, sin ro/1
